simulink model "doubleFM"  (Simulink 9.0)
settings: Solver=FixedStepDiscrete  StartTime=0.0  StopTime=inf  RelTol=1e-3
PreLoadFcn:
  | setenv('MW_MINGW64_LOC','C:\TDM-GCC-64')
StartFcn:
  | tic
StopFcn:
  | toc;
undefined symbols (not defined in the file): fdesignblkfcn, gcbh, magnitude
libraries: dsparch4 x4, UN_HIL_Lib x2, dspobslib x1
Description:
  | QPSK Transmitter and Receiver.
  | 
  | This model shows the implementation of a QPSK transmitter and receiver.
settings Model: FPTRunName=Active  Creator=The MathWorks Inc.  LastModifiedBy=minel
settings DataIOCC: LimitDataPoints=on  SignalLoggingSaveFormat=ModelDataLogs  SaveOutput=off  SaveTime=off
settings OptimizationCC: BooleanDataType=off  DefaultParameterBehavior=Inlined  ExpressionDepthLimit=2147483647  LocalBlockOutputs=off
settings DebuggingCC: AlgebraicLoopMsg=error  SolverPrmCheckMsg=warning  SingleTaskRateTransMsg=error  ParameterPrecisionLossMsg=none  FcnCallInpInsideContextMsg=warning  StateNameClashWarn=warning
settings HardwareCC: TargetBitPerPointer=64  TargetBitPerSizeT=64  TargetBitPerPtrDiffT=64  TargetLongLongMode=on  TargetIntDivRoundTo=Zero  TargetEndianess=LittleEndian  TargetWordSize=64  TargetHWDeviceType=Generic->MATLAB Host Computer  ProdEqTarget=off
settings GRTTargetCC: GeneratePreprocessorConditionals=Disable all
settings ConfigComp: CovSFcnEnable=off
settings SimEventsCC: propDiagStatOutput=1  propPreventDuplicateEvents=0

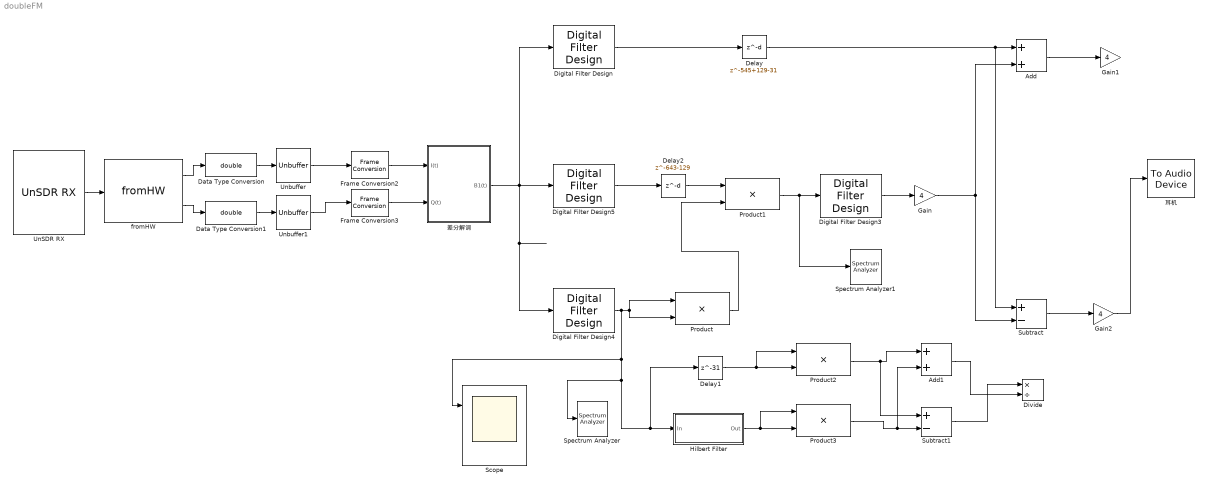
== system doubleFM ==
  Add : Sum
  Add1 : Sum
  Data Type Conversion : DataTypeConversion  OutDataTypeStr=double
  Data Type Conversion1 : DataTypeConversion  OutDataTypeStr=double
  Delay : Delay  DelayLength=545+129-31  InitialCondition=0
  Delay1 : Delay  DelayLength=31  InitialCondition=0
  Delay2 : Delay  DelayLength=643-129  InitialCondition=0
  Digital Filter Design{,3..5} (4 alike) : dsparch4/Digital Filter Design  mwdsp_browser_bugfix_var=off
  Divide : Product  Inputs=*/
  Frame Conversion2 : FrameConversion  InheritSamplingMode=off  OutFrame=Sample-based
  Frame Conversion3 : FrameConversion  InheritSamplingMode=off  OutFrame=Sample-based
  Gain : Gain  Gain=4
  Gain1 : Gain  Gain=4
  Gain2 : Gain  Gain=4
  Hilbert Filter : Subsystem  DialogController=fdesignblkfcn  DialogControllerArgs=DataTag5  InitFcn=fdesignblkfcn(gcbh, {'InitFcn'});  mask(Hilbert Filter){}
      mask help: Design a Hilbert filter
      settings: CopyFcn=fdesignblkfcn(gcbh, {'CopyFcn'});
      mask Help: helpview(mapfilelocation('dsp'), 'dsphilbertfilter');
      mask Display: disp('Hilbert')
  Product{,1..3} (4 alike) : Product
  Scope : Scope  NumInputPorts=2
  Spectrum Analyzer : SpectrumAnalyzer
  Spectrum Analyzer1 : SpectrumAnalyzer
  Subtract : Sum  Inputs=+-
  Subtract1 : Sum  Inputs=+-
  UnSDR RX : UN_HIL_Lib/UnSDR RX  SystemSampleTime=-1
      settings: SourceProductName=HIL Blockset
  Unbuffer : Unbuffer
  Unbuffer1 : Unbuffer
  fromHW : UN_HIL_Lib/fromHW  sp=1/128e3
      settings: SourceProductName=HIL Blockset
  差分解调 : Subsystem
  耳机 : dspobslib/To Audio Device  deviceName=扬声器/听筒 (Realtek Audio)  inheritSampleRate=on  sampleRate=44100  deviceDatatype=Determine from input data type  autoBufferSize=on  bufferSize=4096  queueDuration=2  defaultOutputChannelMapping=on  outputChannelMapping=1:2  outputNumUnderrunSamples=off
      settings: SourceProductName=DSP System Toolbox  SourceProductBaseCode=DS
  wires:
  Unbuffer/1 -> Frame Conversion2/1
  fromHW/1 -> Data Type Conversion/1
  Data Type Conversion/1 -> Unbuffer/1
  fromHW/2 -> Data Type Conversion1/1
  Data Type Conversion1/1 -> Unbuffer1/1
  Unbuffer1/1 -> Frame Conversion3/1
  Frame Conversion2/1 -> 差分解调/1(I(t))
  Frame Conversion3/1 -> 差分解调/2(Q(t))
  UnSDR RX/1 -> fromHW/1
  差分解调/1(B1(t)) -> Digital Filter Design4/1, Digital Filter Design5/1, Digital Filter Design/1
  Digital Filter Design4/1 -> Scope/1, Spectrum Analyzer/1, Delay1/1, Hilbert Filter/1(In), Product/1, Product/2
  Digital Filter Design5/1 -> Delay2/1
  Product1/1 -> Spectrum Analyzer1/1, Digital Filter Design3/1
  Digital Filter Design3/1 -> Gain/1
  Gain/1 -> Add/2, Subtract/2
  Digital Filter Design/1 -> Delay/1
  Subtract/1 -> Gain2/1
  Add/1 -> Gain1/1
  Delay/1 -> Subtract/1, Add/1
  Delay1/1 -> Product2/1, Product2/2
  Hilbert Filter/1(Out) -> Product3/1, Product3/2
  Product2/1 -> Subtract1/1, Add1/1
  Product3/1 -> Add1/2, Subtract1/2
  Subtract1/1 -> Divide/1
  Add1/1 -> Divide/2
  ? -> Scope/2
  Delay2/1 -> Product1/1
  Product/1 -> Product1/2
  Gain2/1 -> 耳机/1

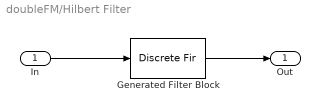
== system doubleFM/Hilbert Filter ==
  In : Inport
  Generated Filter Block : DiscreteFir  Tag=BlockMethodSubSystem  Coefficients=[-0.026449858259791379 -0.00578355491829027 -0.016572261903348456 -0.0095390561131982743 -0.022461390535071568 -0.014999256435125952 -0.030323967074738556 -0.023012528163449009 -0.041429315821655127 -0.035762828939278346 -0.05911752381753177 -0.059034685410808696 -0.094459906652176406 -0.11739830204172252 -0.21797718993610349 -0.62869353747279177 0.62869353747279177 0.21797718993610349 0.11739830204172252 0.094459906652176406 0.059034685410808696 0.05911752381753177 0.035762828939278346 0.041429315821655127 0.023012528163449009 0.030323967074738556 0.014999256435125952 0.022461390535071568 0.0095390561131982743 0.016572261903348456 0.00578355491829027 0.026449858259791379]  InputProcessing=Columns as channels (frame based)
  Out : Outport
  wires:
  Generated Filter Block/1 -> Out/1
  In/1 -> Generated Filter Block/1

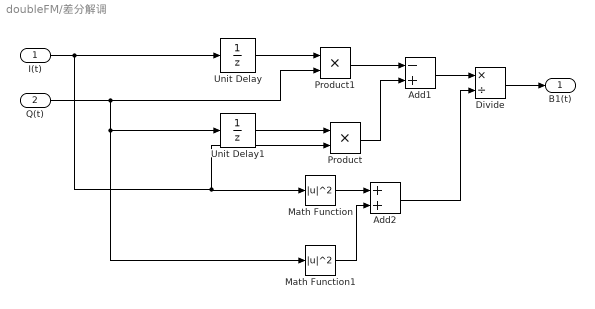
== system doubleFM/差分解调 ==
  I(t) : Inport
  Q(t) : Inport  Port=2
  Add1 : Sum  Inputs=-+
  Add2 : Sum
  Divide : Product  Inputs=*/
  Math Function : Math  Operator=magnitude^2  SaturateOnIntegerOverflow=on
  Math Function1 : Math  Operator=magnitude^2  SaturateOnIntegerOverflow=on
  Product : Product  RndMeth=Zero
  Product1 : Product  RndMeth=Zero
  Unit Delay : UnitDelay  SampleTime=-1
  Unit Delay1 : UnitDelay  SampleTime=-1
  B1(t) : Outport
  wires:
  Add1/1 -> Divide/1
  Add2/1 -> Divide/2
  Product/1 -> Add1/2
  Product1/1 -> Add1/1
  Unit Delay/1 -> Product1/1
  Unit Delay1/1 -> Product/1
  Q(t)/1 -> Math Function1/1, Unit Delay1/1, Product1/2
  I(t)/1 -> Product/2, Math Function/1, Unit Delay/1
  Math Function/1 -> Add2/1
  Math Function1/1 -> Add2/2
  Divide/1 -> B1(t)/1
